simulink model "d_wtfr"  (Simulink 5.1)
settings: Solver=ode45  StartTime=0.0  StopTime=10.0  RelTol=1e-3
libraries: fm_lib x3
settings Model: Creator=fmilano  LastModifiedBy=fmilano  ExtModeAutoUpdateStatusClock=off  SignalLoggingName=logsout  BooleanDataType=on  RTWOptions="-aEnforceIntegerDowncast=1 -aFoldNonRolledExpr=1 -aInlineInvariantSignals=1 -aInlineParameters=0 -aLocalBlockOutputs=1 -aRollThreshold=5 -aZeroInternalMemoryAtStartup=1 -aZeroExternalMemoryAtStartup=1 -aInitFltsAndDblsToZero=1 -aForceBlockIOInitOptimize=0 -aGenerateReport=0 -aGenCodeOnly=0 -aRTWVerbose=1 -aIncludeHyperlinkInReport=0 -aLaunchReport=0 -aGenerateTraceInfo=0  -aForceParamTrailComments=0 -aGenerateComments=1 -aIgnoreCustomStorageClasses=1 -aIncHierarchyInIds=0 -aMaxRTWIdLen=31 -aShowEliminatedStatements=0 -aIncDataTypeInIds=0 -aInsertBlockDesc=0 -aIgnoreTestpoints=0 -aSimulinkBlockComments=1 -aInlinedPrmAccess=\"Literals\"  -aSuppressErrorStatus=0 -aModelReferenceCompliant=1 -aParenthesesLevel=\"Nominal\" -aModelStepFunctionPrototypeControlCompliant=0 -aPortableWordSizes=0 -aParMdlRefBuildCompliant=1 -aSupportNonInlinedSFcns=1 -aSupportContinuousTime=1 -aSupportComplex=1 -aSupportNonFinite=1 -aSupportAbsoluteTime=1 -aMultiwordLength=2048 -aTargetPreCompLibLocation=\"\" -aTargetLibSuffix=\"\" -aTargetFunctionLibrary=\"ANSI_C\" -aTargetFcnLib=\"ansi_tfl_tmw.mat\" -aMultiInstanceERTCode=0 -aLogVarNameModifier=\"rt_\" -aERTFirstTimeCompliant=0 -aIsPILTarget=0 -aCombineOutputUpdateFcns=0 -aGenerateASAP2=0 -aGenerateClassInterface=0 -aGenerateTestInterfaces=0 -aGenerateSampleERTMain=0 -aGenerateFullHeader=1 -aUtilityFuncGeneration=\"Auto\" -aIncludeFileDelimiter=\"Auto\" -aIncludeMdlTerminateFcn=1 -aPurelyIntegerCode=0 -aAutosarCompliant=0 -aERTCustomFileBanners=0 -aRTWCAPIStates=0 -aRTWCAPIParams=0 -aRTWCAPISignals=0 -aMatFileLogging=1 -aCompOptLevelCompliant=1 -aCPPClassGenCompliant=0 -aExtModeIntrfLevel=\"Level1\" -aExtModeMexFile=\"ext_comm\" -aExtModeTransport=0 -aExtModeStaticAllocSize=1000000 -aExtModeTesting=0 -aExtModeStaticAlloc=0 -aExtMode=0 -aERTMultiwordLength=256 -aERTMultiwordTypeDef=\"System defined\"  -aGenerateTraceInfo=0 -aGenerateTraceInfo=0 -aGenerateTraceInfo=0 -aGenerateTraceInfo=0 -aGenerateASAP2=0 -aRTWCAPIStates=0 -aRTWCAPIParams=0 -aRTWCAPISignals=0 -aExtModeIntrfLevel=\"Level1\" -aExtModeMexFile=\"ext_comm\" -aExtModeTransport=0 -aExtModeStaticAllocSize=1000000 -aExtModeTesting=0 -aExtModeStaticAlloc=0 -aExtMode=0"

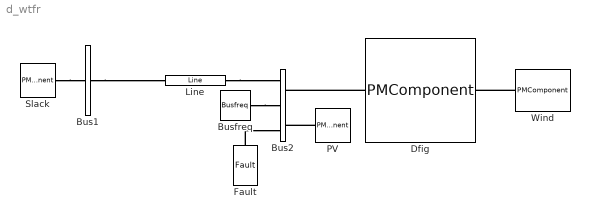
== system d_wtfr ==
  Bus1 : PMComponent  Tag=PSATblock  Description=Connection  PhysicalDomain=psatdomain  LeftPortType=p1  RightPortType=p1  LConnTagsString=__newl0  RConnTagsString=__newr0  mask(Bus){in=1, out=1, p2q=400, p3_4q=[1.00   0.00], p5q=1, p6q=1}
      mask prompts: in "Number of inputs:"; out "Number of outputs:"; p2q "Voltage Rating [kV]"; p3_4q "Voltage initial guess [p.u.   rad]"; p5q "Area number"; p6q "Region number"
      mask help: Bus block
      mask init:
      | fm_inout
      mask CallbackString: ||||fm_block|
      mask Display: plot([0 1 1 0 0],[0 0 1 1 0])
  Bus2 : PMComponent  Tag=PSATblock  Description=Connection  PhysicalDomain=psatdomain  LeftPortType=p1  RightPortType=p1  LConnTagsString=__newl0|__newl1|__newl2  RConnTagsString=__newr0|__newr1  mask(Bus){in=3, out=2, p2q=400, p3_4q=[1.00   0.00], p5q=1, p6q=1}
      mask prompts: in "Number of inputs:"; out "Number of outputs:"; p2q "Voltage Rating [kV]"; p3_4q "Voltage initial guess [p.u.   rad]"; p5q "Area number"; p6q "Region number"
      mask help: Bus block
      mask init:
      | fm_inout
      mask CallbackString: ||||fm_block|
      mask Display: plot([0 1 1 0 0],[0 0 1 1 0])
  Busfreq : fm_lib/Measurements/Busfreq  Tag=PSATblock  Description=Measurements  Orientation=left  PhysicalDomain=psatdomain  SubClassName=unknown  LeftPortType=p1  RightPortType=p1  LConnTagsString=__newl0  p2q=0.001  p3q=0.001  p4q=on
  Dfig : PMComponent  Tag=PSATblock  Description=Wind Turbines  Orientation=left  PhysicalDomain=psatdomain  LeftPortType=p1  RightPortType=p1  LConnTagsString=__newl0  RConnTagsString=__newr0  mask(Dfig){p3_4_5q=[10   400   60], p6_7q=[0.01  0.10], p8_9q=[0.01  0.08], p10q=3.00, p11q=3, p12_13q=[10 3], p14q=10, p15q=0.01, p17_19q=[4 1/89], p16_18q=[75.00  3], p20_21q=[1.00  0.00], p22_23q=[0.7  -0.7], p24q=1, p25q=on}
      mask prompts: p3_4_5q "Power, Voltage and Frequency Ratings [MVA, kV, Hz]"; p6_7q "Stator Resistance Rs and Reactance Xs [p.u.  p.u.]"; p8_9q "Rotor Resitance Rr and Reactance Xr [p.u. p.u.]"; p10q "Magnetization Reactance Xm [p.u.]"; p11q "Inertia Constants Hm  [kWs/kVA]"; p12_13q "Pitch control gain and time constant  Kp, Tp [p.u.  s]"; p14q "Voltage control gain Kv [p.u.]"; p15q "Power Control time constant Te [s]"; p17_19q "Number of poles p and gear box ratio [int  -]"; p16_18q "Blade length and number [m int]"; p20_21q "Pmax and Pmin [p.u.  p.u.]"; p22_23q "Qmax and Qmin [p.u.  p.u.]"; p24q "Number of wind generators that compose the park"; p25q "Connected"
      mask help: This block defines a variable speed wind turbine with doubly fed induction generator.
      mask init:
      | [x,y] = fm_draw('circle');
      | [xh,yh] = fm_draw('helix');
      mask CallbackString: |||||||||||||fm_block
      mask Display:
      | plot(1.4*x,1.4*y,[0,-2],[0 0],[-2 -3 -3 -2 -2],[-1 -1 1 1 -1],[-3 -5],[0 0],[1.4 3.5],[0 0],1,4.35,[0 0 1.075],[-1 -3.25 -3.25],[2.05  2.05],[0 -2.15])
      | plot(1.5*[0.3 0.3]+2.5,0.5*[-1.7 2.7]-3.5,1.5*[ -0.95  -0.95]+2.5,0.5*[-1.7 2.7]-3.5,1.5*[0 0.2]+2.5,0.5*[0.5 0.5]-3.5)
      | plot(1.5*[0.3 -0.95]+2.5,0.5*[2.7 2.7]-3.5,1.5*[0.3 -0.95]+2.5,0.5*[-1.7 -1.7]-3.5)
      | color('blue')
      | plot(x,y)
      | color('cyan')
      | plot(xh-4,3*yh)
      | color('magenta')
      | plot(1.5*[0 0]+2.5,0.5*[-0.5 1.5]-3.5,1.5*[0 -0.2]+2.5,0.5*[-0.5 -0.5]-3.5,1.5*[0 -0.65]+2.5,0.5*[1.5 1.5]-3.5)
      | plot(1.5*[-0.2 -0.2]+2.5,0.5*[-1 0]-3.5,1.5*[-0.2 -0.45]+2.5,0.5*[-1 -0.5]-3.5,1.5*[-0.2 -0.45]+2.5,0.5*[0 -0.5]-3.5,1.5*[-0.45 -0.45]+2.5,0.5*[-1 0]-3.5)
      | plot(1.5*[-0.2 -0.2]+2.5,0.5*[2 1]-3.5,1.5*[-0.45 -0.45]+2.5,0.5*[2 1]-3.5,1.5*[-0.45 -0.2]+2.5,0.5*[2 1.5]-3.5,1.5*[-0.45 -0.2]+2.5,0.5*[1 1.5]-3.5)
      | plot(1.5*[-0.65 -0.65]+2.5,0.5*[-0.5 1.5]-3.5,1.5*[-0.45 -0.65]+2.5,0.5*[-0.5 -0.5]-3.5,1.5*[-0.45 -0.65]+2.5,0.5*[1.5 1.5]-3.5)
      | plot(1.5*[-0.65 -0.85]+2.5,0.5*[0.5 0.5]-3.5,1.5*[-0.3 -0.3]+2.5,0.5*[1.7 2.2]-3.5,1.5*[-0.325 -0.275]+2.5,0.5*[1.975 1.975]-3.5)
  Fault : fm_lib/Faults &  Breakers/Fault  Tag=PSATblock  Description=Faults & Breakers  Orientation=down  PhysicalDomain=psatdomain  SubClassName=unknown  LeftPortType=p1  RightPortType=p1  LConnTagsString=__newl0  p2_3_4q="[100  400  60]"  p5q=1.00  p6q=1.20  p7q=1e-3  p8q=1e-1
  Line : fm_lib/Power Flow/Line  Tag=PSATblock  Description=Power Flow  PhysicalDomain=psatdomain  SubClassName=unknown  LeftPortType=p1  RightPortType=p1  LConnTagsString=__newl0  RConnTagsString=__newr0  p3_4_5q="[100  400  60]"  p6q=0  p8q=0.01  p9q=0.10  p10q=1e-3  p13_14_15q="[0.0  0.0  0.0]"  p16q=on
  PV : PMComponent  Tag=PSATblock  Description=Power Flow  Orientation=left  PhysicalDomain=psatdomain  LeftPortType=p1  RightPortType=p1  RConnTagsString=__newr0  mask(PV){p2_3q=[2  400], p4q=0.8, p5q=1.00, p6_7q=[0.8  -0.2], p8_9q=[1.1  0.9], p10q=1, p11q=on}
      mask prompts: p2_3q "Power and Voltage Ratings [MVA, kV]"; p4q "Active Power [p.u.]"; p5q "Voltage Magnitude [p.u.]"; p6_7q "Qmax and Qmin [p.u.  p.u.]"; p8_9q "Vmax and Vmin [p.u.  p.u.]"; p10q "Loss Participation Factor"; p11q "Connected"
      mask help:
      | This block defines a PV bus for load flow studies:
      |
      | P = Pcost.
      | V = Vdes.
      mask init:
      | [x,y] = fm_draw('circle');
      | [xp,yp] = fm_draw('P');
      mask CallbackString: ||||||fm_block
      mask Display:
      | plot(x,y)
      | color('blue')
      | plot(0.3*xp-0.35,0.6*yp,[0.1 0.3 0.5],[0.3 -0.3 0.3])
  Slack : PMComponent  Tag=PSATblock  Description=Power Flow  PhysicalDomain=psatdomain  LeftPortType=p1  RightPortType=p1  RConnTagsString=__newr0  mask(SW){p2_3q=[100  400], p4q=1.00, p5q=0.00, p6_7q=[1.5  -1.5], p8_9q=[1.1  0.9], p10q=0.80, p11q=1, p12q=on, p13q=on}
      mask prompts: p2_3q "Power and Voltage Ratings [MVA, kV]"; p4q "Voltage Magnitude [p.u.]"; p5q "Reference Phase Angle [rad]"; p6_7q "Qmax and Qmin [p.u.  p.u.]"; p8_9q "Vmax and Vmin  [p.u.  p.u.]"; p10q "Active Power Guess [p.u.]"; p11q "Loss Participation Factor"; p12q "Reference bus"; p13q "Connected"
      mask help:
      | This block defines a V-theta bus:
      |
      | V = V_des
      | theta = theta_des
      mask init:
      | [x,y] = fm_draw('circle');
      | [xt,yt] = fm_draw('theta');
      mask CallbackString: |||||||fm_block|fm_block
      mask Display: plot([0 1 1 0 0],[0 0 1 1 0]), color('blue'), plot([0 1],[0 1],[0 1],[1 0],[0.5 1 0.5 0 0.5],[0 0.5 1 0.5 0])
  Wind : PMComponent  Tag=PSATblock  Description=Wind Turbines  Orientation=left  PhysicalDomain=psatdomain  LeftPortType=p1  RightPortType=p1  RConnTagsString=__newr0  mask(Wind){out=1, p1q=measurements, p2q=15.00, p3q=1.225, p4q=4, p5q=0.1, p6_7q=[20  2], p8_9_10q=[5  15  1], p11_12_13q=[5  15  1], p14_15_16_17q=[50  0.01  0.2  50]}
      mask prompts: out "Number of output ports"; p1q "Wind model type"; p2q "Nominal wind speed [m/s]"; p3q "Air density rho [kg/m^3]"; p4q "Filter time constant tau [s]"; p5q "Sample time for wind measures [s]"; p6_7q "Weibull distribution constants  C and K"; p8_9_10q "Wind ramp constants Tsr, Ter and Awr [s s m/s]"; p11_12_13q "Wind gust constants Tsg, Teg and Awg [s s m/s]"; p14_15_16_17q "Wind turbolence constants h, z0, df and n [m - Hz int]"
      mask help: This block defines wind models for use with wind turbines.
      mask init:
      | fm_inout
      | [xa,ya] = fm_draw('arrow');
      mask StyleString: edit,popup(measurements|weibull|composite),edit,edit,edit,edit,edit,edit,edit,edit
      mask Display:
      | color('cyan')
      | plot(xa,ya,xa-0.2,ya-0.2,xa+0.2,ya+0.2,xa+0.4,ya+0.4,xa-0.4,ya-0.4)
  connections:
  Bus1/RConn1 -- Line/LConn1
  Line/RConn1 -- Bus2/LConn1
  Slack/RConn1 -- Bus1/LConn1
  PV/RConn1 -- Bus2/RConn2
  Wind/RConn1 -- Dfig/LConn1
  Dfig/RConn1 -- Bus2/RConn1
  Busfreq/LConn1 -- Bus2/LConn2
  Fault/LConn1 -- Bus2/LConn3
